simulink model "L1_4R_B_C"  (R2026a)
settings: Solver=VariableStepAuto  StopTime=60
undefined symbols (not defined in the file or in its folder): magnitude
libraries: fl_lib x7, nesl_utility x3, ee_lib x2, eeRmsMeasurement x2, eePowerMeasurement x1
settings Model: Creator=andre  LastModifiedBy=andre

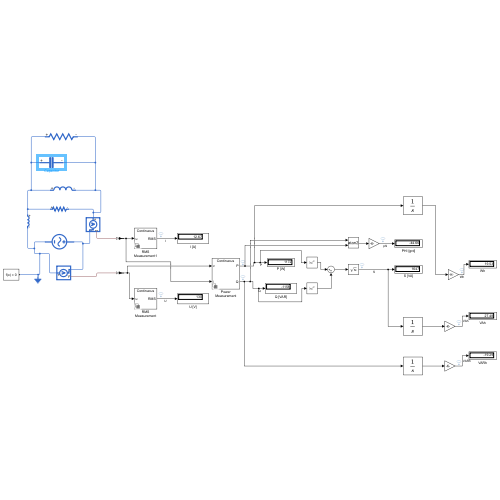
[thumbnail: Simulink's stored preview of the top-level diagram]
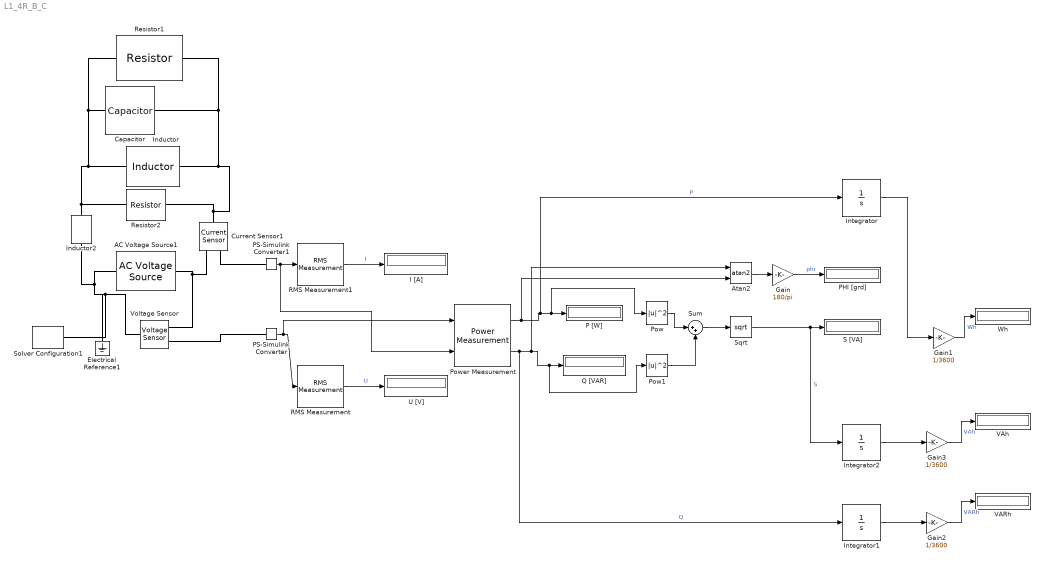
== system L1_4R_B_C ==
  AC Voltage Source1 : fl_lib/Electrical/Electrical Sources/AC Voltage Source  amp=130*sqrt(2) V  shift=0 deg  frequency=50 Hz
  Atan2 : Trigonometry  Operator=atan2
  Capacitor : fl_lib/Electrical/Electrical Elements/Capacitor  c=33 uF  r=0.5 Ohm  g=0 1/Ohm  i_specify=off  i_priority=None  i=0 A  i_nominal_specify=off  i_nominal_value=1  i_nominal_unit=A  v_specify=off  v_priority=None  v=0 V  v_nominal_specify=off  v_nominal_value=1  v_nominal_unit=V  vc_specify=off  vc_priority=High  vc=0 V  vc_nominal_specify=off  vc_nominal_value=1  vc_nominal_unit=V
  Current Sensor1 : fl_lib/Electrical/Electrical Sensors/Current Sensor
  Electrical Reference1 : fl_lib/Electrical/Electrical Elements/Electrical Reference
  Gain : Gain  Gain=180/pi
  Gain1 : Gain  Gain=1/3600
  Gain2 : Gain  Gain=1/3600
  Gain3 : Gain  Gain=1/3600
  I [A] : Display
  Inductor : ee_lib/Passive/Inductor  l=257.38 mH  enable_L_tol=ee.enum.toleranceApplication.none  L_tol=20  tol_distribution=ee.enum.toleranceDistribution.uniform  nSigma=4  r=21.5 Ohm  g=1e-9 1/Ohm  enable_operating_limits=ee.enum.enable.no  operating_limit_action=ee.enum.passive.reportOpLim.warn  max_working_current=1 A  power_rating=1 W  i_L_specify=off  i_L_priority=High  i_L=0 A  i_L_nominal_specify=off  i_L_nominal_value=1  i_L_nominal_unit=A
  Inductor2 : ee_lib/Passive/Inductor  l=0.00069 H  enable_L_tol=ee.enum.toleranceApplication.none  L_tol=20  tol_distribution=ee.enum.toleranceDistribution.uniform  nSigma=4  r=0 Ohm  g=1e-9 1/Ohm  enable_operating_limits=ee.enum.enable.no  operating_limit_action=ee.enum.passive.reportOpLim.warn  max_working_current=1 A  power_rating=1 W  i_L_specify=off  i_L_priority=High  i_L=0 A  i_L_nominal_specify=off  i_L_nominal_value=1  i_L_nominal_unit=A
  Integrator : Integrator
  Integrator1 : Integrator
  Integrator2 : Integrator
  P [W] : Display
  PHI [grd] : Display
  PS-Simulink Converter : nesl_utility/PS-Simulink Converter  PhysicalDomain=network_engine_domain  SubClassName=ps_output  LeftPortType=input  RightPortType=output  PseudoPeriodic=off  Frequencies=[]  VectorFormat=inherit  Unit=inherit  AffineConversion=off
  PS-Simulink Converter1 : nesl_utility/PS-Simulink Converter  PhysicalDomain=network_engine_domain  SubClassName=ps_output  LeftPortType=input  RightPortType=output  PseudoPeriodic=off  Frequencies=[]  VectorFormat=inherit  Unit=inherit  AffineConversion=off
  Pow : Math  Operator=magnitude^2  SignedPower=on  RndMeth=Zero
  Pow1 : Math  Operator=magnitude^2  SignedPower=on  RndMeth=Zero
  Power Measurement : eePowerMeasurement/Power Measurement  LabelModeActiveChoice=Continuous  F=50  K=1  Ts=0
  Q [VAR] : Display
  RMS Measurement : eeRmsMeasurement/RMS Measurement  LabelModeActiveChoice=Total  F=50  SpecifyHarmonics=off  K=[0 1 2]  Ts=0
      settings: LibrarySourceBlock=|
      | ee_sl_lib/Measurements/RMS
      | Measurement
  RMS Measurement1 : eeRmsMeasurement/RMS Measurement  LabelModeActiveChoice=Total  F=50  SpecifyHarmonics=off  K=[0 1 2]  Ts=0
      settings: LibrarySourceBlock=|
      | ee_sl_lib/Measurements/RMS
      | Measurement
  Resistor1 : fl_lib/Electrical/Electrical Elements/Resistor  R=81 Ohm  i_specify=off  i_priority=None  i=0 A  i_nominal_specify=off  i_nominal_value=1  i_nominal_unit=A  v_specify=off  v_priority=None  v=0 V  v_nominal_specify=off  v_nominal_value=1  v_nominal_unit=V
  Resistor2 : fl_lib/Electrical/Electrical Elements/Resistor  R=121 Ohm  i_specify=off  i_priority=None  i=0 A  i_nominal_specify=off  i_nominal_value=1  i_nominal_unit=A  v_specify=off  v_priority=None  v=0 V  v_nominal_specify=off  v_nominal_value=1  v_nominal_unit=V
  S [VA] : Display
  Solver Configuration1 : nesl_utility/Solver Configuration  PhysicalDomain=network_engine_domain  SubClassName=solver  LeftPortType=input  RightPortType=generic  Tones=[]  Harmonics=[]  SimulateNoise=off  Profile=off  UseLocalSampling=off  EnableSwitchedLinearOptims=on  FrequencyDomain=off  UseCCode=off  RelTol=0.001  AbsTol=0.001  MinStep=1e-09  ToWorkspace=off  RevertToSquareIcSolve=off  NumHomotopyIterations=100  PhasorMode=off  PhasorModeNumHarmonics=1  ConsistencySolver=NEWTON_XTOL_AFTER_FTOL  CanonicalOrdering=CANONICAL  OptimizeIntermediates=OPTIMIZED  IndexReductionMethod=DerivativeReplacement  DoDC=off  ResidualTolerance=1e-09  ConsistencyTolSource=GLOBAL  ConsistencyAbsTol=0.001  ConsistencyRelTol=0.001  ConsistencyTolFactor=0.001  UseLocalSolver=off  LocalSolverChoice=NE_BACKWARD_EULER_ADVANCER  ResolveIndetEquations=on  FunctionEvalNumThread=1  LocalSolverSampleTime=0.001  DoFixedCost=off  MaxNonlinIter=3  MaxModeIter=2  ComputeImpulses=off  ImpulseIterations=2  LinearAlgebra=auto  LinearAlgebraNumThread=0  EquationFormulation=NE_TIME_EF  DelaysMemoryBudget=1024  AutomaticFiltering=on  FilteringTimeConstant=0.001  PartitionStorageMethod=AS_NEEDED  PartitionMemoryBudget=1024  PartitionMethod=ROBUST  MultibodyUseLocalSolver=off  MultibodyLocalSolverChoice=ODE1  MultibodyLocalSolverSampleTime=0.001
  Sqrt : Sqrt
  Sum : Sum  Inputs=|++
  U [V] : Display
  VARh : Display
  VAh : Display
  Voltage Sensor : fl_lib/Electrical/Electrical Sensors/Voltage Sensor
  Wh : Display
  wires:
  PS-Simulink Converter1/1 -> Power Measurement/2, RMS Measurement1/1
  RMS Measurement1/1 -> I [A]/1  "I"
  RMS Measurement/1 -> U [V]/1  "U"
  Power Measurement/1 -> Atan2/2, Integrator/1, Pow/1, P [W]/1  "P"
  Power Measurement/2 -> Integrator1/1, Atan2/1, Pow1/1, Q [VAR]/1  "Q"
  PS-Simulink Converter/1 -> Power Measurement/1, RMS Measurement/1
  Pow/1 -> Sum/1
  Pow1/1 -> Sum/2
  Sum/1 -> Sqrt/1
  Atan2/1 -> Gain/1
  Gain/1 -> PHI [grd]/1  "phi"
  Integrator/1 -> Gain1/1
  Gain1/1 -> Wh/1  "Wh"
  Integrator1/1 -> Gain2/1
  Gain2/1 -> VARh/1  "VARh"
  Integrator2/1 -> Gain3/1
  Sqrt/1 -> Integrator2/1, S [VA]/1  "S"
  Gain3/1 -> VAh/1  "VAh"
  connections:
  Voltage Sensor/LConn1 -- Electrical Reference1/LConn1 -- Solver Configuration1/RConn1 -- Inductor2/RConn1 -- AC Voltage Source1/RConn1
  Voltage Sensor/RConn2 -- Current Sensor1/RConn2 -- AC Voltage Source1/LConn1
  Current Sensor1/RConn1 -- PS-Simulink Converter1/LConn1
  Voltage Sensor/RConn1 -- PS-Simulink Converter/LConn1
  Resistor1/RConn1 -- Inductor/RConn1 -- Resistor2/RConn1 -- Current Sensor1/LConn1 -- Capacitor/RConn1
  Resistor1/LConn1 -- Capacitor/LConn1 -- Inductor2/LConn1 -- Resistor2/LConn1 -- Inductor/LConn1
